simulink model "sampleModel1752_2_sub_sub_sub"  (R2023a)
settings: Solver=VariableStepAuto  StartTime=0.0  StopTime=10.0  RelTol=1e-3
libraries: simulink x2, hdlsllib x2
settings Model: Creator=user1  LastModifiedBy=user1
settings OptimizationCC: BlockReduction=off  ConditionallyExecuteInputs=off

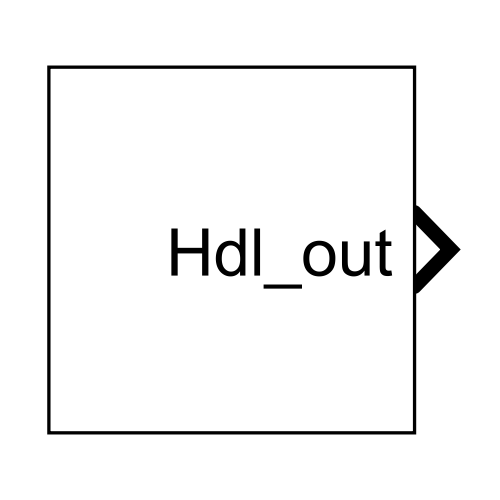
[thumbnail: Simulink's stored preview of the top-level diagram]
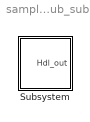
== system sampleModel1752_2_sub_sub_sub ==
  Subsystem : Subsystem

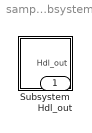
== system sampleModel1752_2_sub_sub_sub/Subsystem ==
  Subsystem : Subsystem
  Hdl_out : Outport  OutDataTypeStr=uint8

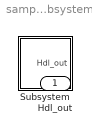
== system sampleModel1752_2_sub_sub_sub/Subsystem/Subsystem ==
  Subsystem : Subsystem
  Hdl_out : Outport  OutDataTypeStr=uint8

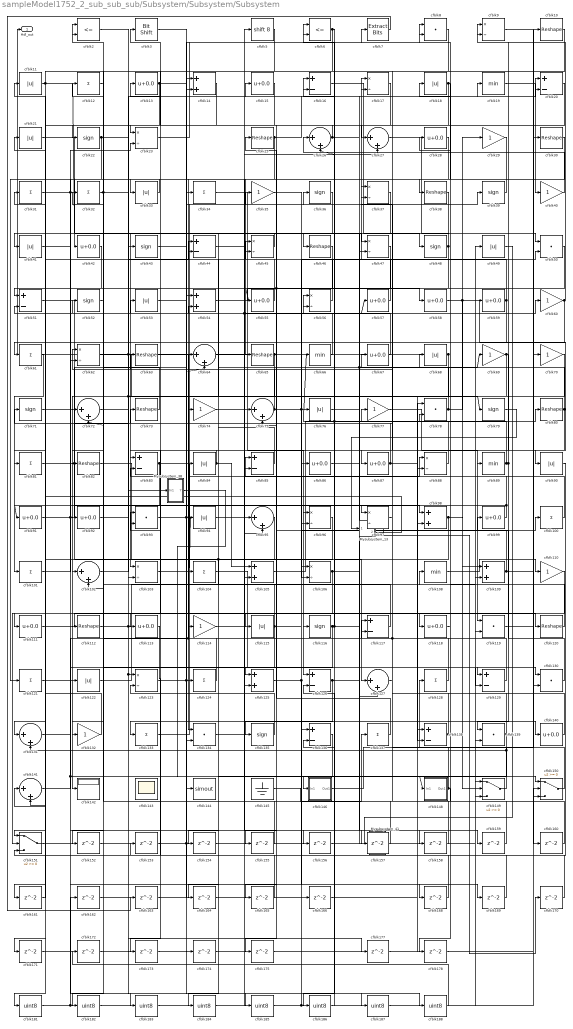
== system sampleModel1752_2_sub_sub_sub/Subsystem/Subsystem/Subsystem ==
  Mysubsystem_13 : Subsystem  TreatAsAtomicUnit=on  RTWFcnName=Mysubsystem_13
      settings: RTWFcnNameOpts=User specified  RTWFileNameOpts=Use function name
  Mysubsystem_38 : Subsystem  TreatAsAtomicUnit=on  RTWFcnName=Mysubsystem_38
      settings: RTWFcnNameOpts=User specified  RTWFileNameOpts=Use function name
  Mysubsystem_41 : Subsystem  TreatAsAtomicUnit=on  RTWFcnName=Mysubsystem_41
      settings: RTWFcnNameOpts=User specified  RTWFileNameOpts=Use function name
  cfblk{10,25,30,38,46,63,65,73,80,82,112,120} (12 alike) : Reshape
  cfblk{12,31..32,34,61,81,100..101,104,121,124,128,133,137} (14 alike) : Sum  Inputs=+  OutDataTypeStr=uint8
  cfblk{26..27,64,72,75,95,102,127,131,141} (10 alike) : Sum  Inputs=|++  OutDataTypeStr=uint8
  cfblk{9,17,23,37,45,47,56,62,88,96..97,103,106,123} (14 alike) : Product  Inputs=*/  OutDataTypeStr=uint8  RndMeth=Zero  SaturateOnIntegerOverflow=on
  cfblk{14,54,98,105,109,125} (6 alike) : Sum  OutDataTypeStr=uint8
  cfblk{19,66,89,108} (4 alike) : MinMax  OutDataTypeStr=uint8
  cfblk{11,18,21,33,41,49,53,68,76,84,90,94,115,122} (14 alike) : Abs  OutDataTypeStr=uint8  SaturateOnIntegerOverflow=off
  cfblk{29,35,40,60,69..70,74,77,110,114,132} (11 alike) : Gain  OutDataTypeStr=uint8
  cfblk{13,15,28,42,55,57..59,67,86..87,91..92,99,111,113,118,140} (18 alike) : Bias  Bias=0.0  SaturateOnIntegerOverflow=off
  cfblk{22,36,39,43,48,52,71,79,116,135} (10 alike) : Signum
  cfblk{16,20,44,51,83,85,117,126,129,136,138} (11 alike) : Sum  Inputs=+-  OutDataTypeStr=uint8
  cfblk{8,50,78,93,119,130,134,139} (8 alike) : DotProduct  OutDataTypeStr=uint8
  cfblk142 : Display
  cfblk143 : Scope
      settings: Floating=on
  cfblk144 : ToWorkspace  VariableName=simout  SaveFormat=Timeseries  SampleTime=-1
  cfblk145 : Ground
  cfblk146 : Subsystem
      settings: LibrarySourceBlock=|
      | hdlsllib/Ports &
      | Subsystems/Subsystem
  cfblk148 : Subsystem
      settings: LibrarySourceBlock=|
      | hdlsllib/Ports &
      | Subsystems/Subsystem
  cfblk149 : Switch  OutDataTypeStr=uint8  SaturateOnIntegerOverflow=off  InputSameDT=off
  cfblk150 : Switch  OutDataTypeStr=uint8  SaturateOnIntegerOverflow=off  InputSameDT=off
  cfblk151 : Switch  OutDataTypeStr=uint8  SaturateOnIntegerOverflow=off  InputSameDT=off
  cfblk{152..166,168..175,177..178} (25 alike) : Delay  SampleTime=1
  cfblk{181..188} (8 alike) : DataTypeConversion  OutDataTypeStr=uint8  SaturateOnIntegerOverflow=off  RndMeth=Floor
  cfblk2 : RelationalOperator  Operator=<=  OutDataTypeStr=boolean  InputSameDT=off
  cfblk3 : hdlsllib/Logic and Bit Operations/Bit Shift  mode=Shift Left Logical  N=0
  cfblk5 : ArithShift  BitShiftNumber=8
  cfblk6 : RelationalOperator  Operator=<=  OutDataTypeStr=boolean  InputSameDT=off
  cfblk7 : simulink/Logic and Bit Operations/Extract Bits  bitsToExtract=Upper half  numBits=8  bitIdxRange=[0 7]  outScalingMode=Preserve fixed-point scaling
      settings: LibrarySourceBlock=|
      | hdlsllib/Logic and Bit
      | Operations/Extract Bits
  Hdl_out : Outport  OutDataTypeStr=uint8
  wires:
  cfblk61/1 -> cfblk101/1
  cfblk88/1 -> cfblk26/2, cfblk66/1
  cfblk132/1 -> cfblk31/1
  cfblk133/1 -> cfblk108/1
  cfblk118/1 -> cfblk85/1
  cfblk38/1 -> cfblk103/1
  cfblk149/1 -> cfblk131/2, cfblk128/1
  cfblk99/1 -> cfblk56/2, cfblk91/1
  cfblk105/1 -> cfblk80/1
  cfblk16/1 -> cfblk48/1
  cfblk33/1 -> cfblk121/1
  cfblk82/1 -> cfblk127/1
  cfblk66/1 -> cfblk11/1
  cfblk57/1 -> cfblk17/1
  cfblk28/1 -> cfblk134/1
  cfblk14/1 -> cfblk111/1
  cfblk47/1 -> cfblk135/1
  cfblk111/1 -> cfblk118/1
  cfblk63/1 -> cfblk36/1
  cfblk68/1 -> Hdl_out/1, cfblk134/2
  cfblk34/1 -> cfblk126/1
  cfblk11/1 -> cfblk61/1, cfblk42/1
  cfblk87/1 -> cfblk129/2, cfblk73/1
  cfblk21/1 -> cfblk86/1
  cfblk35/1 -> cfblk106/1
  cfblk151/1 -> cfblk75/1, cfblk124/1, cfblk64/2
  cfblk51/1 -> cfblk97/1
  cfblk93/1 -> cfblk35/1, cfblk88/1
  cfblk104/1 -> cfblk130/1
  cfblk65/1 -> cfblk175/1, cfblk142/1
  cfblk117/1 -> cfblk2/1
  cfblk83/1 -> cfblk132/1, cfblk106/2
  cfblk98/1 -> cfblk149/2, cfblk146/1(In1)
  cfblk126/1 -> cfblk173/1, cfblk20/2, cfblk69/1
  cfblk75/1 -> cfblk50/2, cfblk62/1
  cfblk78/1 -> cfblk29/1, cfblk53/1
  cfblk62/1 -> cfblk44/2, cfblk144/1
  cfblk54/1 -> cfblk58/1
  cfblk70/1 -> cfblk96/1
  cfblk58/1 -> cfblk109/1, cfblk90/1
  cfblk20/1 -> cfblk27/1
  cfblk52/1 -> cfblk102/1
  cfblk27/1 -> cfblk50/1
  cfblk60/1 -> cfblk161/1, cfblk9/1
  cfblk128/1 -> cfblk93/1
  cfblk42/1 -> cfblk51/1
  cfblk138/1 -> cfblk78/2, cfblk71/1
  cfblk67/1 -> cfblk52/1
  cfblk77/1 -> cfblk119/1
  cfblk110/1 -> cfblk151/1
  cfblk103/1 -> cfblk39/1
  cfblk56/1 -> cfblk21/1
  cfblk124/1 -> cfblk32/1, cfblk64/1
  cfblk106/1 -> cfblk68/1, cfblk151/2
  cfblk32/1 -> cfblk72/2, Mysubsystem_38/1(In1)
  cfblk10/1 -> cfblk81/1
  cfblk64/1 -> cfblk138/2
  cfblk96/1 -> cfblk154/1, cfblk141/2
  cfblk23/1 -> cfblk7/1
  cfblk37/1 -> cfblk115/1
  cfblk36/1 -> cfblk74/1
  cfblk120/1 -> cfblk18/1
  cfblk140/1 -> cfblk28/1
  cfblk145/1 -> cfblk137/1
  cfblk8/1 -> cfblk87/1
  cfblk6/1 -> cfblk186/1, cfblk82/1
  cfblk81/1 -> cfblk104/1, cfblk14/1
  cfblk122/1 -> cfblk59/1
  cfblk113/1 -> cfblk133/1
  cfblk112/1 -> cfblk177/1, cfblk84/1
  cfblk136/1 -> cfblk184/1
  cfblk48/1 -> cfblk131/1, cfblk46/1
  cfblk125/1 -> cfblk168/1, cfblk100/1
  cfblk129/1 -> cfblk37/2, cfblk94/1
  cfblk102/1 -> cfblk15/1
  cfblk17/1 -> cfblk75/2
  cfblk46/1 -> cfblk103/2
  cfblk73/1 -> cfblk12/1
  cfblk135/1 -> cfblk3/1
  cfblk29/1 -> cfblk65/1
  cfblk141/1 -> cfblk148/1(In1), cfblk122/1
  cfblk95/1 -> cfblk181/1
  cfblk39/1 -> cfblk33/1
  cfblk150/1 -> cfblk117/1
  cfblk19/1 -> cfblk40/1
  cfblk59/1 -> cfblk112/1, cfblk13/1
  cfblk84/1 -> cfblk105/1, cfblk83/1
  cfblk45/1 -> cfblk41/1
  cfblk89/1 -> cfblk6/2, cfblk9/2, cfblk139/1
  cfblk31/1 -> cfblk183/1, cfblk127/2
  cfblk69/1 -> cfblk89/1, cfblk116/1
  cfblk2/1 -> cfblk47/1
  cfblk108/1 -> cfblk110/1
  cfblk22/1 -> cfblk62/2, cfblk79/1, cfblk188/1, cfblk123/1
  cfblk123/1 -> cfblk130/2
  cfblk40/1 -> cfblk26/1
  cfblk100/1 -> cfblk16/1
  cfblk121/1 -> cfblk114/1
  cfblk92/1 -> cfblk129/1
  cfblk86/1 -> cfblk120/1
  cfblk71/1 -> cfblk34/1
  cfblk85/1 -> cfblk54/2
  cfblk55/1 -> cfblk45/1
  cfblk116/1 -> cfblk165/1, cfblk56/1, cfblk19/1
  cfblk119/1 -> cfblk10/1
  cfblk80/1 -> cfblk113/1, cfblk6/1
  cfblk72/1 -> cfblk16/2
  cfblk30/1 -> cfblk102/2
  cfblk5/1 -> cfblk23/1
  cfblk25/1 -> cfblk105/2, cfblk17/2
  cfblk114/1 -> cfblk140/1
  cfblk137/1 -> cfblk25/1
  cfblk12/1 -> cfblk72/1
  cfblk13/1 -> cfblk92/1, cfblk8/1
  cfblk130/1 -> cfblk99/1
  cfblk148/1(Out1) -> cfblk178/1, cfblk37/1
  cfblk3/1 -> cfblk98/1
  cfblk146/1(Out1) -> cfblk30/1
  cfblk26/1 -> cfblk20/1, cfblk22/1
  cfblk18/1 -> cfblk38/1, cfblk125/1, cfblk55/1
  cfblk139/1 -> cfblk164/1, cfblk63/1
  cfblk134/1 -> cfblk27/2
  cfblk115/1 -> cfblk182/1, cfblk44/1, cfblk60/1, cfblk76/1
  cfblk127/1 -> cfblk67/1
  cfblk109/1 -> cfblk45/2, cfblk70/1
  cfblk101/1 -> cfblk23/2
  cfblk74/1 -> cfblk57/1, cfblk5/1
  cfblk97/1 -> cfblk77/1
  cfblk91/1 -> cfblk125/2, cfblk43/1
  cfblk15/1 -> cfblk152/1
  cfblk152/1 -> cfblk47/2
  cfblk90/1 -> cfblk153/1
  cfblk153/1 -> cfblk149/1
  cfblk154/1 -> cfblk97/2
  cfblk50/1 -> cfblk155/1
  cfblk155/1 -> cfblk2/2
  cfblk131/1 -> cfblk156/1
  cfblk156/1 -> cfblk98/2
  cfblk94/1 -> cfblk157/1
  cfblk157/1 -> cfblk54/1
  cfblk76/1 -> cfblk158/1
  cfblk158/1 -> cfblk93/2
  cfblk44/1 -> cfblk159/1
  cfblk159/1 -> cfblk117/2
  cfblk9/1 -> cfblk160/1
  cfblk160/1 -> cfblk8/2
  cfblk161/1 -> cfblk141/1
  cfblk162/1 -> cfblk14/2
  cfblk7/1 -> cfblk163/1
  cfblk163/1 -> cfblk88/2
  cfblk164/1 -> cfblk85/2
  cfblk165/1 -> cfblk151/3
  cfblk166/1 -> cfblk126/2
  cfblk168/1 -> cfblk83/2
  cfblk41/1 -> cfblk169/1
  cfblk169/1 -> cfblk123/2
  cfblk170/1 -> cfblk51/2
  cfblk171/1 -> cfblk119/2
  cfblk173/1 -> cfblk96/2
  cfblk53/1 -> cfblk174/1
  cfblk174/1 -> cfblk78/1
  cfblk175/1 -> cfblk149/3
  cfblk177/1 -> cfblk109/2
  cfblk178/1 -> cfblk150/2
  cfblk181/1 -> cfblk139/2, cfblk162/1
  cfblk182/1 -> cfblk95/1
  cfblk183/1 -> cfblk95/2
  cfblk184/1 -> cfblk49/1, cfblk166/1
  cfblk43/1 -> cfblk185/1
  cfblk185/1 -> cfblk136/1
  cfblk186/1 -> cfblk136/2
  cfblk172/1 -> cfblk187/1
  cfblk187/1 -> cfblk150/3
  cfblk188/1 -> cfblk172/1
  cfblk79/1 -> Mysubsystem_13/1(In1)
  Mysubsystem_13/1(Out1) -> cfblk170/1
  Mysubsystem_13/2(Out2) -> cfblk171/1
  Mysubsystem_38/1(Y) -> cfblk150/1
  cfblk49/1 -> Mysubsystem_41/1(In1)
  Mysubsystem_41/1(Out1) -> cfblk138/1

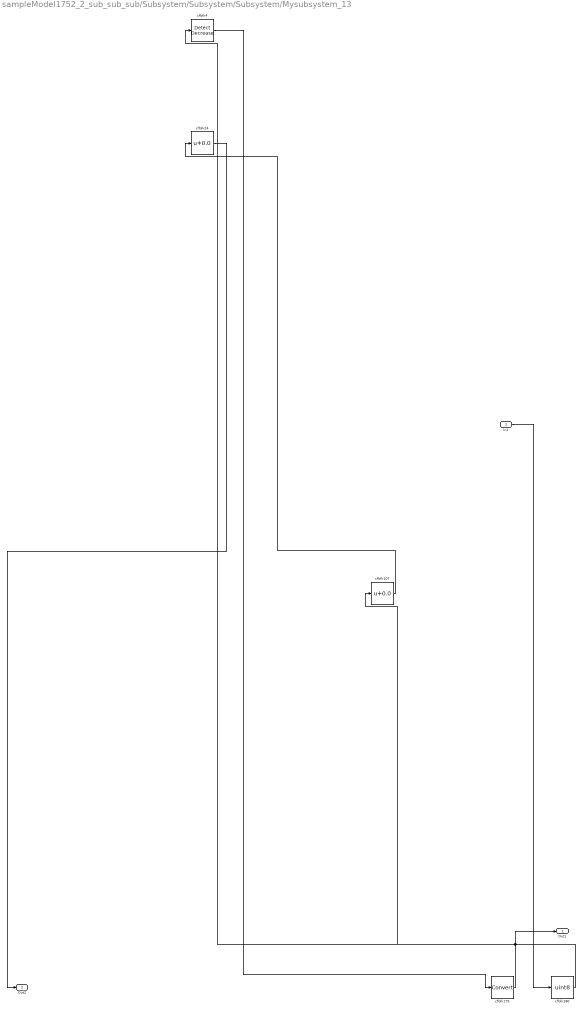
== system sampleModel1752_2_sub_sub_sub/Subsystem/Subsystem/Subsystem/Mysubsystem_13 ==
  In1 : Inport
  cfblk107 : Bias  Bias=0.0  SaturateOnIntegerOverflow=off
  cfblk179 : DataTypeConversion  SaturateOnIntegerOverflow=off  RndMeth=Floor
  cfblk180 : DataTypeConversion  OutDataTypeStr=uint8  SaturateOnIntegerOverflow=off  RndMeth=Floor
  cfblk24 : Bias  Bias=0.0  SaturateOnIntegerOverflow=off
  cfblk4 : simulink/Logic and Bit Operations/Detect Decrease  vinit=0.0  OutDataTypeStr=boolean
      settings: LibrarySourceBlock=|
      | hdlsllib/Logic and Bit
      | Operations/Detect
      | Decrease
  Out1 : Outport
  Out2 : Outport  Port=2
  wires:
  In1/1 -> cfblk180/1
  cfblk180/1 -> cfblk4/1
  cfblk179/1 -> cfblk107/1, Out1/1
  cfblk24/1 -> Out2/1
  cfblk107/1 -> cfblk24/1
  cfblk4/1 -> cfblk179/1

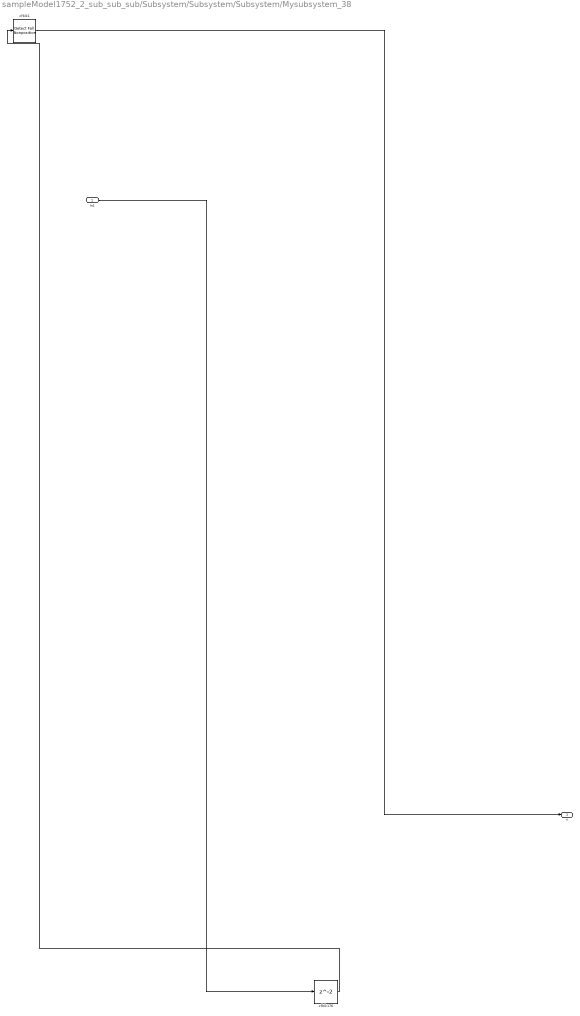
== system sampleModel1752_2_sub_sub_sub/Subsystem/Subsystem/Subsystem/Mysubsystem_38 ==
  In1 : Inport
  cfblk1 : hdlsllib/Logic and Bit Operations/Detect Fall Nonpositive  vinit=0  OutDataTypeStr=boolean
  cfblk176 : Delay  SampleTime=1
  Y : Outport
  wires:
  cfblk1/1 -> Y/1
  cfblk176/1 -> cfblk1/1
  In1/1 -> cfblk176/1

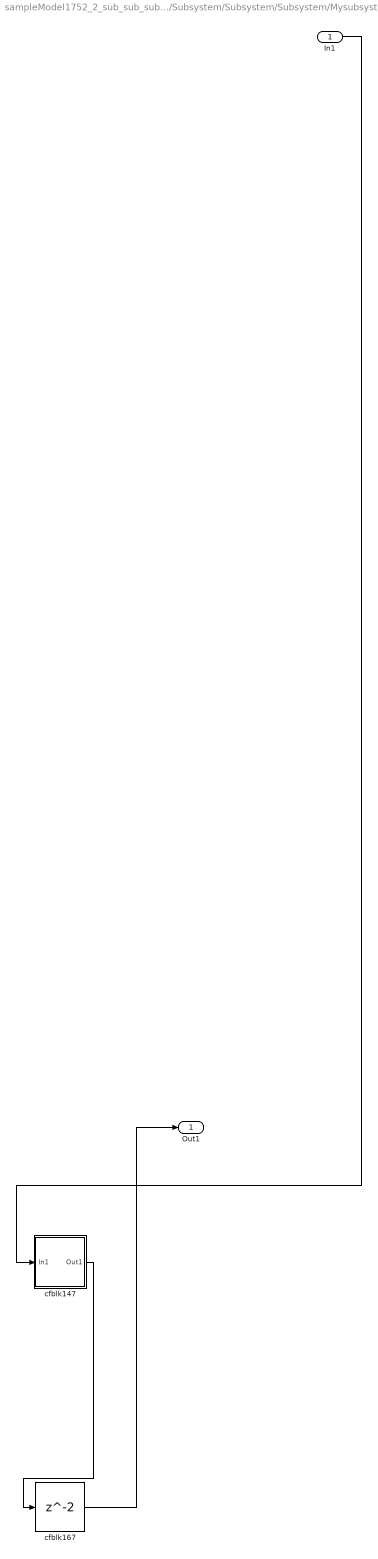
== system sampleModel1752_2_sub_sub_sub/Subsystem/Subsystem/Subsystem/Mysubsystem_41 ==
  In1 : Inport
  cfblk147 : Subsystem
      settings: LibrarySourceBlock=|
      | hdlsllib/Ports &
      | Subsystems/Subsystem
  cfblk167 : Delay  SampleTime=1
  Out1 : Outport
  wires:
  In1/1 -> cfblk147/1(In1)
  cfblk167/1 -> Out1/1
  cfblk147/1(Out1) -> cfblk167/1

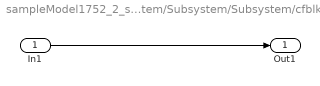
== system sampleModel1752_2_sub_sub_sub/Subsystem/Subsystem/Subsystem/cfblk146 ==
  In1 : Inport
  Out1 : Outport
  wires:
  In1/1 -> Out1/1

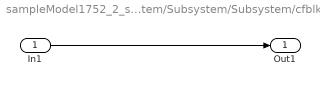
== system sampleModel1752_2_sub_sub_sub/Subsystem/Subsystem/Subsystem/cfblk148 ==
  In1 : Inport
  Out1 : Outport
  wires:
  In1/1 -> Out1/1

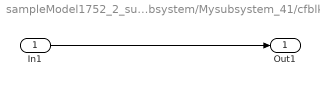
== system sampleModel1752_2_sub_sub_sub/Subsystem/Subsystem/Subsystem/Mysubsystem_41/cfblk147 ==
  In1 : Inport
  Out1 : Outport
  wires:
  In1/1 -> Out1/1
